simulink model "Target_Control_System"  (R2021b)
settings: Solver=FixedStepDiscrete  StartTime=0.0  StopTime=5  RelTol=1e-3
PreLoadFcn:
  | RTWConfigurationCB('preloadfcn', bdroot);
PostLoadFcn:
  | load('configuration/data_struct.mat');
  | load('configuration/fluxMaps_propMotor.mat');
  | load('configuration/parameterInit_PROP.mat');
  | load('configuration/parameterInit_PUMP.mat');
  | load('configuration/parameterInit_PITCH.mat');
  | load('configuration/parameterInit_TILT.mat');
  | %load('configuration/base_workspace_signal_definition.mat');
  | %load('resolvedatastores_to_baseworkspace_for_faster_simulation.mat');
model workspace (MAT data in the model file):
  SIMULATION_OPTIONS : Simulink.Parameter (value not decoded)
  TARGET_CODE_GEN : Simulink.Parameter (value not decoded)
  TCS_SAMPLE_FREQ_HZ : Simulink.Parameter (value not decoded)
symbols that are objects in the model workspace (value not decoded): TARGET_CODE_GEN, TCS_SAMPLE_FREQ_HZ
undefined symbols (not defined in the file): A_DQ_REF_LPF_INIT__PITCH, A_DQ_REF_LPF_INIT__PROP, A_DQ_REF_LPF_INIT__PUMP, A_DQ_REF_LPF_INIT__TILT, A_OBSERVER_CONFIDENCE_INIT__PITCH, A_OBSERVER_CONFIDENCE_INIT__PROP, A_OBSERVER_CONFIDENCE_INIT__PUMP, A_OBSERVER_CONFIDENCE_INIT__TILT, ACTUATOR_MAX_ANGLE_TRIP__PITCH, ACTUATOR_MIN_ANGLE_TRIP__PITCH, ACTUATOR_POS_SENSOR_INV_DIRECTION__PITCH, ACTUATOR_POS_SENSOR_INV_DIRECTION__TILT, ACTUATOR_POS_SENSOR_OFFSET__PITCH, ACTUATOR_POS_SENSOR_OFFSET__TILT, ADC_scaler1_baseaddr_TILT, ADC_SCALER_FLOAT_TO_FIXPOINT_EXPANSION, ANGLE_ELEC_FROM_SENSOR_OFFSET_INIT__PITCH, ANGLE_ELEC_FROM_SENSOR_OFFSET_INIT__PROP, ANGLE_ELEC_FROM_SENSOR_OFFSET_INIT__PUMP, ANGLE_ELEC_FROM_SENSOR_OFFSET_INIT__TILT, AUTO_CLEAR_FAULTS_ENABLED__PITCH, AUTO_CLEAR_FAULTS_ENABLED__PROP, AUTO_CLEAR_FAULTS_ENABLED__PUMP, AUTO_CLEAR_FAULTS_ENABLED__TILT, AUTO_CLEAR_FAULTS_WAIT_TICKS__PITCH, AUTO_CLEAR_FAULTS_WAIT_TICKS__PROP, AUTO_CLEAR_FAULTS_WAIT_TICKS__PUMP, AUTO_CLEAR_FAULTS_WAIT_TICKS__TILT, AUTO_I_ZERO_IDLE_TICKS__PITCH, AUTO_I_ZERO_IDLE_TICKS__PROP, AUTO_I_ZERO_IDLE_TICKS__PUMP, AUTO_I_ZERO_IDLE_TICKS__TILT, AUTO_I_ZERO_OFFSET_IDC_THRESHOLD__PITCH, AUTO_I_ZERO_OFFSET_IDC_THRESHOLD__PROP, AUTO_I_ZERO_OFFSET_IDC_THRESHOLD__PUMP, AUTO_I_ZERO_OFFSET_IDC_THRESHOLD__TILT, AUTO_I_ZERO_OFFSET_IPH_THRESHOLD__PITCH, AUTO_I_ZERO_OFFSET_IPH_THRESHOLD__PROP, AUTO_I_ZERO_OFFSET_IPH_THRESHOLD__PUMP, AUTO_I_ZERO_OFFSET_IPH_THRESHOLD__TILT, AUTO_SENSORLESS_SWITCHOVER_DISABLE_OMEGA, AUTO_SENSORLESS_SWITCHOVER_ENABLE_OMEGA, AUTO_SENSORLESS_SWITCHOVER_MIN_CONFIDENCE, AUXILIARY_PROTECTION_UNIT_BASEADDR__TILT, blanking_max_error_omega_INIT_PITCH, blanking_max_error_omega_INIT_TILT, blanking_max_error_position_INIT_PITCH, blanking_max_error_position_INIT_TILT, BRUTE_START_I_Q_REF_RAMP_SPEED__PITCH, BRUTE_START_I_Q_REF_RAMP_SPEED__PROP, BRUTE_START_I_Q_REF_RAMP_SPEED__PUMP, BRUTE_START_I_Q_REF_RAMP_SPEED__TILT, CONTROL_LOOP_DT_INIT__PITCH, CONTROL_LOOP_DT_INIT__PROP, CONTROL_LOOP_DT_INIT__PUMP, CONTROL_LOOP_DT_INIT__TILT, CORRECTION_FILTER_SCALE__PITCH, CORRECTION_FILTER_SCALE__PROP, CORRECTION_FILTER_SCALE__PUMP, CORRECTION_FILTER_SCALE__TILT ... (+458)
libraries: simulink x178, Reusables_Lib x24
(part 14 of 47)

== system Target_Control_System/Target_Control_System/MainLoop/propMotor_mainLoop/motorTaskMainFastStep(&oProp)/Lowpass Filtered Quantities for External World - Prop ==
  note: Low-pass filtered quantities for external world
  lpfQuantities : TriggerPort  TriggerType=function-call  VariantControl=Variant
  Constant1 : Constant  Value=0.00008  OutDataTypeStr=single  SampleTime=-1
  Data Store Read17 : DataStoreRead  DataStoreName=oProp  DataStoreElements=oProp.oMot_.oIn_.fId_  IndexOptions=Index vector (dialog)  Indices=1  OutputSizes=1
  Data Store Read18 : DataStoreRead  DataStoreName=oProp  DataStoreElements=oProp.oMot_.oIn_.fIq_  IndexOptions=Index vector (dialog)  Indices=1  OutputSizes=1
  Data Store Read19 : DataStoreRead  DataStoreName=oProp  DataStoreElements=oProp.oMot_.oIn_.fTEstimate_  IndexOptions=Index vector (dialog)  Indices=1  OutputSizes=1
  Data Store Read20 : DataStoreRead  DataStoreName=oProp  DataStoreElements=oProp.oMot_.oOut_.fPowerDcLpf_  IndexOptions=Index vector (dialog)  Indices=1  OutputSizes=1
  Data Store Read21 : DataStoreRead  DataStoreName=oProp  DataStoreElements=oProp.oMot_.oOut_.fPowerDcXlpf_  IndexOptions=Index vector (dialog)  Indices=1  OutputSizes=1
  Data Store Read22 : DataStoreRead  DataStoreName=oProp  DataStoreElements=oProp.oMot_.oIn_.fOmegaEObserverLpf2_  IndexOptions=Index vector (dialog)  Indices=1  OutputSizes=1
  Data Store Read23 : DataStoreRead  DataStoreName=oProp  DataStoreElements=oProp.oMot_.oOut_.fOmegaEObserverXlpf2_  IndexOptions=Index vector (dialog)  Indices=1  OutputSizes=1
  Data Store Read24 : DataStoreRead  DataStoreName=oProp  DataStoreElements=oProp.oMot_.oParam_.fAOmegaXfilter2_  IndexOptions=Index vector (dialog)  Indices=1  OutputSizes=1
  Data Store Read27 : DataStoreRead  DataStoreName=oProp  DataStoreElements=oProp.oMot_.oParam_.fSlowPassFactor_  IndexOptions=Index vector (dialog)  Indices=1  OutputSizes=1
  Data Store Read28 : DataStoreRead  DataStoreName=oProp  DataStoreElements=oProp.oMot_.oIn_.fIPhaseMagnitude_  IndexOptions=Index vector (dialog)  Indices=1  OutputSizes=1
  Data Store Read29 : DataStoreRead  DataStoreName=oProp  DataStoreElements=oProp.oMot_.oState_.fIPhaseMagnitudeLpf_  IndexOptions=Index vector (dialog)  Indices=1  OutputSizes=1
  Data Store Read43 : DataStoreRead  DataStoreName=oProp  DataStoreElements=oProp.oMot_.oOut_.fIdLpf_  IndexOptions=Index vector (dialog)  Indices=1  OutputSizes=1
  Data Store Read44 : DataStoreRead  DataStoreName=oProp  DataStoreElements=oProp.oMot_.oOut_.fIqLpf_  IndexOptions=Index vector (dialog)  Indices=1  OutputSizes=1
  Data Store Read45 : DataStoreRead  DataStoreName=oProp  DataStoreElements=oProp.oMot_.oIn_.oAdcData_.fUdc_  IndexOptions=Index vector (dialog)  Indices=1  OutputSizes=1
  Data Store Read46 : DataStoreRead  DataStoreName=oProp  DataStoreElements=oProp.oMot_.oOut_.fUdcLpf_  IndexOptions=Index vector (dialog)  Indices=1  OutputSizes=1
  Data Store Read47 : DataStoreRead  DataStoreName=oProp  DataStoreElements=oProp.oMot_.oIn_.oAdcData_.fIdc_  IndexOptions=Index vector (dialog)  Indices=1  OutputSizes=1
  Data Store Read48 : DataStoreRead  DataStoreName=oProp  DataStoreElements=oProp.oMot_.oOut_.fIdcLpf_  IndexOptions=Index vector (dialog)  Indices=1  OutputSizes=1
  Data Store Read49 : DataStoreRead  DataStoreName=oProp  DataStoreElements=oProp.oMot_.oIn_.fPowerDc_  IndexOptions=Index vector (dialog)  Indices=1  OutputSizes=1
  Data Store Read50 : DataStoreRead  DataStoreName=oProp  DataStoreElements=oProp.oMot_.oOut_.fPowerDcLpf_  IndexOptions=Index vector (dialog)  Indices=1  OutputSizes=1
  Data Store Read52 : DataStoreRead  DataStoreName=oProp  DataStoreElements=oProp.oMot_.oOut_.fTEstimateLpf_  IndexOptions=Index vector (dialog)  Indices=1  OutputSizes=1
  Data Store Read53 : DataStoreRead  DataStoreName=oProp  DataStoreElements=oProp.oMot_.oState_.oRampDataIqRef_.fRampOut_  IndexOptions=Index vector (dialog)  Indices=1  OutputSizes=1
  Data Store Read54 : DataStoreRead  DataStoreName=oProp  DataStoreElements=oProp.oMot_.oOut_.fIqRefRampOutLpf_  IndexOptions=Index vector (dialog)  Indices=1  OutputSizes=1
  Data Store Read55 : DataStoreRead  DataStoreName=oProp  DataStoreElements=oProp.oMot_.oParam_.fADqRefLpf_  IndexOptions=Index vector (dialog)  Indices=1  OutputSizes=1
  Data Store Read56 : DataStoreRead  DataStoreName=oProp  DataStoreElements=oProp.oMot_.oIn_.fIdRefTotal_  IndexOptions=Index vector (dialog)  Indices=1  OutputSizes=1
  Data Store Read57 : DataStoreRead  DataStoreName=oProp  DataStoreElements=oProp.oMot_.oOut_.fIdRefLpf_  IndexOptions=Index vector (dialog)  Indices=1  OutputSizes=1
  Data Store Read58 : DataStoreRead  DataStoreName=oProp  DataStoreElements=oProp.oMot_.oIn_.fUqRef_  IndexOptions=Index vector (dialog)  Indices=1  OutputSizes=1
  Data Store Read59 : DataStoreRead  DataStoreName=oProp  DataStoreElements=oProp.oMot_.oOut_.fUqRefLpf_  IndexOptions=Index vector (dialog)  Indices=1  OutputSizes=1
  Data Store Read60 : DataStoreRead  DataStoreName=oProp  DataStoreElements=oProp.oMot_.oIn_.fUdRef_  IndexOptions=Index vector (dialog)  Indices=1  OutputSizes=1
  Data Store Read62 : DataStoreRead  DataStoreName=oProp  DataStoreElements=oProp.oMot_.oOut_.fUdRefLpf_  IndexOptions=Index vector (dialog)  Indices=1  OutputSizes=1
  Data Store Write2 : DataStoreWrite  DataStoreName=oProp  DataStoreElements=oProp.oMot_.oOut_.fPowerDcXlpf_  IndexOptions=Index vector (dialog)  Indices=1  OutputSizes=1
  Data Store Write20 : DataStoreWrite  DataStoreName=oProp  DataStoreElements=oProp.oMot_.oState_.fIPhaseMagnitudeLpf_  IndexOptions=Index vector (dialog)  Indices=1  OutputSizes=1
  Data Store Write21 : DataStoreWrite  DataStoreName=oProp  DataStoreElements=oProp.oMot_.oOut_.fIdLpf_  IndexOptions=Index vector (dialog)  Indices=1  OutputSizes=1
  Data Store Write22 : DataStoreWrite  DataStoreName=oProp  DataStoreElements=oProp.oMot_.oOut_.fIqLpf_  IndexOptions=Index vector (dialog)  Indices=1  OutputSizes=1
  Data Store Write24 : DataStoreWrite  DataStoreName=oProp  DataStoreElements=oProp.oMot_.oOut_.fUdcLpf_  IndexOptions=Index vector (dialog)  Indices=1  OutputSizes=1
  Data Store Write25 : DataStoreWrite  DataStoreName=oProp  DataStoreElements=oProp.oMot_.oOut_.fIdcLpf_  IndexOptions=Index vector (dialog)  Indices=1  OutputSizes=1
  Data Store Write28 : DataStoreWrite  DataStoreName=oProp  DataStoreElements=oProp.oMot_.oOut_.fPowerDcLpf_  IndexOptions=Index vector (dialog)  Indices=1  OutputSizes=1
  Data Store Write29 : DataStoreWrite  DataStoreName=oProp  DataStoreElements=oProp.oMot_.oOut_.fTEstimateLpf_  IndexOptions=Index vector (dialog)  Indices=1  OutputSizes=1
  Data Store Write3 : DataStoreWrite  DataStoreName=oProp  DataStoreElements=oProp.oMot_.oOut_.fOmegaEObserverXlpf2_  IndexOptions=Index vector (dialog)  Indices=1  OutputSizes=1
  Data Store Write30 : DataStoreWrite  DataStoreName=oProp  DataStoreElements=oProp.oMot_.oOut_.fIqRefRampOutLpf_  IndexOptions=Index vector (dialog)  Indices=1  OutputSizes=1
  Data Store Write31 : DataStoreWrite  DataStoreName=oProp  DataStoreElements=oProp.oMot_.oOut_.fIdRefLpf_  IndexOptions=Index vector (dialog)  Indices=1  OutputSizes=1
  Data Store Write32 : DataStoreWrite  DataStoreName=oProp  DataStoreElements=oProp.oMot_.oOut_.fUqRefLpf_  IndexOptions=Index vector (dialog)  Indices=1  OutputSizes=1
  Data Store Write34 : DataStoreWrite  DataStoreName=oProp  DataStoreElements=oProp.oMot_.oOut_.fUdRefLpf_  IndexOptions=Index vector (dialog)  Indices=1  OutputSizes=1
  Divide{8..20} (13 alike) : Product  Inputs=**
  Sum{4..5,7,10..11,13,15,18,20..22,25,29} (13 alike) : Sum  Inputs=|+-
  Sum{3,6,8..9,12,14,16..17,19,24,26,30..31} (13 alike) : Sum  Inputs=|++
  wires:
  Sum10/1 -> Divide13/2
  Data Store Read22/1 -> Sum22/1
  Divide12/1 -> Sum9/1
  Sum3/1 -> Data Store Write20/1
  Divide20/1 -> Sum24/1
  Sum13/1 -> Divide12/2
  Sum19/1 -> Data Store Write31/1
  Data Store Read46/1 -> Sum13/2, Sum9/2
  Divide17/1 -> Sum30/1
  Data Store Read43/1 -> Sum4/2, Sum6/2
  Sum18/1 -> Divide15/2
  Sum22/1 -> Divide18/2
  Data Store Read23/1 -> Sum26/2, Sum22/2
  Divide9/1 -> Sum6/1
  Data Store Read24/1 -> Divide18/1
  Data Store Read18/1 -> Sum5/1
  Sum8/1 -> Data Store Write22/1
  Data Store Read44/1 -> Sum5/2, Sum8/2
  Data Store Read28/1 -> Sum7/1
  Data Store Read21/1 -> Sum24/2, Sum21/2
  Sum9/1 -> Data Store Write24/1
  Sum5/1 -> Divide10/2
  Sum4/1 -> Divide9/2
  Data Store Read55/1 -> Divide15/1, Divide16/1, Divide19/1, Divide17/1
  Sum15/1 -> Divide14/2
  Divide8/1 -> Sum3/1
  Sum29/1 -> Divide17/2
  Data Store Read27/1 -> Divide8/1, Divide9/1, Divide10/1, Divide12/1, Divide13/1, Divide14/1, Divide11/1
  Sum11/1 -> Divide11/2
  Sum14/1 -> Data Store Write28/1
  Data Store Read20/1 -> Sum21/1
  Data Store Read54/1 -> Sum18/2, Sum17/2
  Data Store Read56/1 -> Sum20/1
  Divide18/1 -> Sum26/1
  Constant1/1 -> Divide20/1
  Sum30/1 -> Data Store Write32/1
  Data Store Read49/1 -> Sum11/1
  Sum25/1 -> Divide19/2
  Data Store Read45/1 -> Sum13/1
  Divide15/1 -> Sum17/1
  Divide14/1 -> Sum16/1
  Sum26/1 -> Data Store Write3/1
  Sum24/1 -> Data Store Write2/1
  Data Store Read17/1 -> Sum4/1
  Divide13/1 -> Sum12/1
  Sum20/1 -> Divide16/2
  Data Store Read62/1 -> Sum25/2, Sum31/2
  Divide16/1 -> Sum19/1
  Data Store Read60/1 -> Sum25/1
  Data Store Read57/1 -> Sum20/2, Sum19/2
  Sum21/1 -> Divide20/2
  Data Store Read48/1 -> Sum12/2, Sum10/2
  Sum16/1 -> Data Store Write29/1
  Divide11/1 -> Sum14/1
  Data Store Read19/1 -> Sum15/1
  Sum6/1 -> Data Store Write21/1
  Sum7/1 -> Divide8/2
  Data Store Read29/1 -> Sum7/2, Sum3/2
  Data Store Read50/1 -> Sum14/2, Sum11/2
  Divide10/1 -> Sum8/1
  Sum12/1 -> Data Store Write25/1
  Data Store Read59/1 -> Sum29/2, Sum30/2
  Data Store Read47/1 -> Sum10/1
  Data Store Read52/1 -> Sum16/2, Sum15/2
  Sum17/1 -> Data Store Write30/1
  Data Store Read53/1 -> Sum18/1
  Sum31/1 -> Data Store Write34/1
  Divide19/1 -> Sum31/1
  Data Store Read58/1 -> Sum29/1

== system Target_Control_System/Target_Control_System/MainLoop/propMotor_mainLoop/motorTaskMainFastStep(&oProp)/Observer Confidence - Prop ==
  note: Observer confidence
      | // Two contributions, each adding 1/3 to give a value in range 0.0-1.0:
      | 	//  1. Magnitude of estimated flux relative to nominal flux (perhaps not for induction motors)
      | 	//  2. The relative noise on the estimated speed
  observerConfidence : TriggerPort  TriggerType=function-call  VariantControl=Variant
  Abs2 : Abs  OutDataTypeStr=single
  Abs3 : Abs  OutDataTypeStr=single
  Abs5 : Abs  OutDataTypeStr=single
  Add10 : Sum  Inputs=|-+
  Add11 : Sum
  Add2 : Sum  Inputs=+-
  Add7 : Sum  Inputs=|+-
  Add8 : Sum  Inputs=|-+
  Add9 : Sum  Inputs=|-+
  Constant14 : Constant  OutDataTypeStr=single  SampleTime=-1
  Data Store Read1 : DataStoreRead  DataStoreName=oProp  DataStoreElements=oProp.oMot_.oParam_.fAObserverConfidence_  IndexOptions=Index vector (dialog)  Indices=1  OutputSizes=1
  Data Store Read37 : DataStoreRead  DataStoreName=oProp  DataStoreElements=oProp.oMot_.oIn_.fOmegaEObserverLpf2_  IndexOptions=Index vector (dialog)  Indices=1  OutputSizes=1
  Data Store Read4 : DataStoreRead  DataStoreName=oProp  DataStoreElements=oProp.oMot_.oIn_.fFluxMainMagnitudeLpf_  IndexOptions=Index vector (dialog)  Indices=1  OutputSizes=1
  Data Store Read61 : DataStoreRead  DataStoreName=oProp  DataStoreElements=oProp.oMot_.oIn_.fOmegaEObserverRaw2_  IndexOptions=Index vector (dialog)  Indices=1  OutputSizes=1
  Data Store Read83 : DataStoreRead  DataStoreName=oProp  DataStoreElements=oProp.oMot_.oParam_.fMainFluxNominal_  IndexOptions=Index vector (dialog)  Indices=1  OutputSizes=1
  Data Store Write33 : DataStoreWrite  DataStoreName=oProp  DataStoreElements=oProp.oMot_.oState_.fObserverConfidence_  IndexOptions=Index vector (dialog)  Indices=1  OutputSizes=1
  Divide1 : Product  Inputs=*/
  Divide2 : Product  Inputs=*/
  Gain11 : Gain  Gain=0.83
  Gain5 : Gain  Gain=0.4
  Half : Constant  Value=0.5  OutDataTypeStr=single  SampleTime=-1
  Half1 : Constant  Value=0.5  OutDataTypeStr=single  SampleTime=-1
  IIR : Subsystem
  Saturation2 : Saturate  UpperLimit=1.25  LowerLimit=-inf
  Saturation3 : Saturate  UpperLimit=0.6  LowerLimit=-inf
  Switch3 : Switch  Criteria=u2 > Threshold  Threshold=0.5
  Zero8 : Constant  Value=0  OutDataTypeStr=Inherit: Inherit via back propagation  SampleTime=-1
  isNaN : RelationalOperator  Operator=isNaN  OutDataTypeStr=boolean  RndMeth=Simplest
  wires:
  Data Store Read1/1 -> IIR/3(K), Add2/2
  Abs5/1 -> Divide2/2
  Add11/1 -> isNaN/1, Switch3/3  "fObserverConfidence_"
  Data Store Read83/1 -> Divide1/2, Add7/2
  Gain5/1 -> Add8/1
  Add2/1 -> IIR/2(1-K)
  Half1/1 -> Add10/2
  isNaN/1 -> Switch3/2
  Abs3/1 -> Divide2/1
  Gain11/1 -> Add10/1
  Divide1/1 -> Saturation2/1
  Switch3/1 -> IIR/1(In)
  Zero8/1 -> Switch3/1
  Abs2/1 -> Divide1/1
  Data Store Read37/1 -> Add9/2, Abs5/1
  Half/1 -> Add8/2
  Saturation2/1 -> Gain5/1
  Constant14/1 -> Add2/1
  Data Store Read61/1 -> Add9/1
  Add9/1 -> Abs3/1
  Divide2/1 -> Saturation3/1
  IIR/1(Out) -> Data Store Write33/1
  Add7/1 -> Abs2/1
  Add8/1 -> Add11/1
  Add10/1 -> Add11/2
  Saturation3/1 -> Gain11/1
  Data Store Read4/1 -> Add7/1

== system Target_Control_System/Target_Control_System/MainLoop/propMotor_mainLoop/motorTaskMainFastStep(&oProp)/PWM for Simulation ==
  Enable : EnablePort
  Constant : Constant  OutDataTypeStr=uint32  SampleTime=-1
  Constant1 : Constant  Value=0  OutDataTypeStr=uint32  SampleTime=-1
  Data Store Read1 : DataStoreRead  DataStoreName=oProp  DataStoreElements=oProp.oIsr_.oState_.iPwmUpdated_  IndexOptions=Index vector (dialog)  Indices=1  OutputSizes=1
  Data Store Write18 : DataStoreWrite  DataStoreName=oProp  DataStoreElements=oProp.oIsr_.oOut_.uiPwmSetByIsr_  IndexOptions=Index vector (dialog)  Indices=1  OutputSizes=1
  NOT : Logic  Operator=NOT  AllPortsSameDT=off  OutDataTypeStr=boolean
  Scope : Scope
  Subsystem : Subsystem
  Subsystem1 : Subsystem
  Switch1 : Switch  Criteria=u2 > Threshold
  Switch2 : Switch  Criteria=u2 > Threshold
  Motor : Outport
  wires:
  NOT/1 -> Subsystem1/Enable
  Subsystem1/1(propMotor_PWMticks) -> Switch1/3
  Subsystem/1(propMotor_PWMticks) -> Switch1/1
  Constant1/1 -> Switch2/3
  Constant/1 -> Switch2/1
  Switch2/1 -> Data Store Write18/1
  Switch1/1 -> Motor/1  "propMotor_PWMticks"
  Data Store Read1/1 -> Subsystem/Enable, Switch1/2, NOT/1, Scope/1, Switch2/2

== system Target_Control_System/Target_Control_System/MainLoop/propMotor_mainLoop/motorTaskMainFastStep(&oProp)/motorTaskManagePwmRequestFlags() ==
  motorTaskManagePwmRequestFlags : TriggerPort  TriggerType=function-call  VariantControl=Variant
  Constant : Constant  Value=0  OutDataTypeStr=uint32  SampleTime=-1
  Data Store Read : DataStoreRead  DataStoreName=oProp  DataStoreElements=oProp.oMot_.oIn_.uiPwmSetByIsr_  IndexOptions=Index vector (dialog)  Indices=1  OutputSizes=1
  Data Store Read1 : DataStoreRead  DataStoreName=oProp  DataStoreElements=oProp.oMot_.oOut_.uiPwmRequestFromMain_  IndexOptions=Index vector (dialog)  Indices=1  OutputSizes=1
  Data Store Write : DataStoreWrite  DataStoreName=oProp  DataStoreElements=oProp.oMot_.oOut_.uiPwmRequestFromMain_  IndexOptions=Index vector (dialog)  Indices=1  OutputSizes=1
  Switch : Switch  Criteria=u2 > Threshold  OutDataTypeStr=uint32
  wires:
  Data Store Read1/1 -> Switch/3
  Constant/1 -> Switch/1
  Switch/1 -> Data Store Write/1
  Data Store Read/1 -> Switch/2

== system Target_Control_System/Target_Control_System/MainLoop/propMotor_mainLoop/motorTaskMainFastStep(&oProp)/resetFlag_uiDataFromIsrToMainUpdated ==
  resetFlag_uiDataFromIsrToMainUpdated : TriggerPort  TriggerType=function-call  VariantControl=Variant
  Constant : Constant  Value=0  OutDataTypeStr=uint32  SampleTime=-1
  Data Store Write9 : DataStoreWrite  DataStoreName=oProp  DataStoreElements=oProp.oMot_.oIn_.uiDataFromIsrToMainUpdated_  IndexOptions=Index vector (dialog)  Indices=1  OutputSizes=1
  wires:
  Constant/1 -> Data Store Write9/1

== system Target_Control_System/Target_Control_System/MainLoop/pumpMotor_mainLoop/Decimation gate A for 200 Hz Pump/Current offset nulling ==
  note: Try to perform current sensor offset nulling at least once as soon as possible:
      | (Subsequent nulling steps are performed only once the drive has been idle for a while)
  function : TriggerPort  TriggerType=function-call  VariantControl=Variant
  Constant2 : Constant  Value=0  OutDataTypeStr=uint32  SampleTime=-1
  Data Store Read2 : DataStoreRead  DataStoreName=oPump  DataStoreElements=oPump.oMot_.oState_.uiCurrentOffsetNullingPerformed_  IndexOptions=Index vector (dialog)  Indices=1  OutputSizes=1
  GreaterThan1 : RelationalOperator  Operator=>  OutDataTypeStr=boolean  RndMeth=Simplest
  NOT : Logic  Operator=NOT  IconShape=distinctive  AllPortsSameDT=off  OutDataTypeStr=boolean
  initiateOffsetNulling(&oPump) : Subsystem  TreatAsAtomicUnit=on
  wires:
  NOT/1 -> initiateOffsetNulling(&oPump)/Enable
  GreaterThan1/1 -> NOT/1
  Constant2/1 -> GreaterThan1/2
  Data Store Read2/1 -> GreaterThan1/1

== system Target_Control_System/Target_Control_System/MainLoop/pumpMotor_mainLoop/Decimation gate A for 200 Hz Pump/Subsystem ==
  Idle_Controller : TriggerPort  TriggerType=function-call  VariantControl=Variant
  AND7 : Logic  AllPortsSameDT=off  OutDataTypeStr=boolean
  Data Store Read1 : DataStoreRead  DataStoreName=oPump  DataStoreElements=oPump.oMot_.oParam_.oPiDataIdleCtrl_.fState_  IndexOptions=Index vector (dialog)  Indices=1  OutputSizes=1
  Data Store Read2 : DataStoreRead  DataStoreName=oPump  DataStoreElements=oPump.oMot_.oParam_.fRpmBlankingUnblankConfidence_  IndexOptions=Index vector (dialog)  Indices=1  OutputSizes=1
  Data Store Read25 : DataStoreRead  DataStoreName=oPump  DataStoreElements=oPump.oMot_.oState_.uiDriveState_  IndexOptions=Index vector (dialog)  Indices=1  OutputSizes=1
  Data Store Read3 : DataStoreRead  DataStoreName=oPump  DataStoreElements=oPump.oMot_.oParam_.fRpmBlankingBlankConfidence_  IndexOptions=Index vector (dialog)  Indices=1  OutputSizes=1
  Data Store Read32 : DataStoreRead  DataStoreName=oPump  DataStoreElements=oPump.oMot_.oState_.fObserverConfidence_  IndexOptions=Index vector (dialog)  Indices=1  OutputSizes=1
  Data Store Read51 : DataStoreRead  DataStoreName=oPump  DataStoreElements=oPump.oMot_.oState_.uiDriveState_  IndexOptions=Index vector (dialog)  Indices=1  OutputSizes=1
  Data Store Read65 : DataStoreRead  DataStoreName=oPump  DataStoreElements=oPump.oMot_.oOut_.fOmegaEObserverXlpf2_  IndexOptions=Index vector (dialog)  Indices=1  OutputSizes=1
  Data Store Read66 : DataStoreRead  DataStoreName=oPump  DataStoreElements=oPump.oMot_.oState_.fIdleCtrlOmegaEMin_  IndexOptions=Index vector (dialog)  Indices=1  OutputSizes=1
  Data Store Read67 : DataStoreRead  DataStoreName=oPump  DataStoreElements=oPump.oMot_.oParam_.oPiDataIdleCtrl_.oParameter_.fKp_  IndexOptions=Index vector (dialog)  Indices=1  OutputSizes=1
  Data Store Read69 : DataStoreRead  DataStoreName=oPump  DataStoreElements=oPump.oMot_.oParam_.oPiDataIdleCtrl_.oParameter_.fKi_  IndexOptions=Index vector (dialog)  Indices=1  OutputSizes=1
  Data Store Read70 : DataStoreRead  DataStoreName=oPump  DataStoreElements=oPump.oMot_.oParam_.oPiDataIdleCtrl_.oParameter_.fIntMax_  IndexOptions=Index vector (dialog)  Indices=1  OutputSizes=1
  Data Store Read94 : DataStoreRead  DataStoreName=oPump  DataStoreElements=oPump.oMot_.oParam_.oPiDataIdleCtrl_.oParameter_.fOutMax_  IndexOptions=Index vector (dialog)  Indices=1  OutputSizes=1
  Data Store Read95 : DataStoreRead  DataStoreName=oPump  DataStoreElements=oPump.oMot_.oParam_.oPiDataIdleCtrl_.oParameter_.fLoopDt_  IndexOptions=Index vector (dialog)  Indices=1  OutputSizes=1
  Data Store Write5 : DataStoreWrite  DataStoreName=oPump  DataStoreElements=oPump.oMot_.oState_.iRpmBlankingActive_  IndexOptions=Index vector (dialog)  Indices=1  OutputSizes=1
  Equal12 : RelationalOperator  Operator===  OutDataTypeStr=boolean  RndMeth=Simplest
  Equal16 : RelationalOperator  Operator=~=  OutDataTypeStr=boolean  RndMeth=Simplest
  Equal17 : RelationalOperator  Operator=~=  OutDataTypeStr=boolean  RndMeth=Simplest
  NOT : Logic  Operator=NOT  AllPortsSameDT=off  OutDataTypeStr=boolean
  OR (Never blank in state 200)1 : Logic  Operator=OR  AllPortsSameDT=off  OutDataTypeStr=boolean
  Subsystem : Subsystem
  Switch2 : Switch  Criteria=u2 > Threshold  Threshold=0.5  OutDataTypeStr=int32
  Zero18 : Constant  Value=0  OutDataTypeStr=single  SampleTime=-1
  Zero19 : Constant  OutDataTypeStr=single  SampleTime=-1
  Zero8 : Constant  Value=0  OutDataTypeStr=single  SampleTime=-1
  const12 : Constant  Value=200  OutDataTypeStr=uint32  SampleTime=-1
  const13 : Constant  Value=211  OutDataTypeStr=uint32  SampleTime=-1
  const14 : Constant  Value=212  OutDataTypeStr=uint32  SampleTime=-1
  greater1 : RelationalOperator  Operator=>  OutDataTypeStr=boolean  RndMeth=Simplest
  piControllerStep_Idle_Controller : Subsystem  SystemSampleTime=1/200
  smaller1 : RelationalOperator  Operator=<  OutDataTypeStr=boolean  RndMeth=Simplest
  wires:
  smaller1/1 -> Switch2/3
  Switch2/1 -> Data Store Write5/1
  Zero8/1 -> Switch2/1
  Data Store Read32/1 -> smaller1/1, greater1/1
  const12/1 -> Equal12/2
  Data Store Read2/1 -> greater1/2
  Equal12/1 -> OR (Never blank in state 200)1/1
  Data Store Read3/1 -> smaller1/2
  greater1/1 -> OR (Never blank in state 200)1/2
  Data Store Read25/1 -> Equal12/1
  OR (Never blank in state 200)1/1 -> Switch2/2
  NOT/1 -> Subsystem/Enable
  Data Store Read1/1 -> piControllerStep_Idle_Controller/11(fState)
  const13/1 -> Equal16/1
  Data Store Read67/1 -> piControllerStep_Idle_Controller/3(fKp)
  Data Store Read94/1 -> piControllerStep_Idle_Controller/8(fOutMax)
  Data Store Read66/1 -> piControllerStep_Idle_Controller/2(fTarget)
  Zero19/1 -> piControllerStep_Idle_Controller/5(fScale)
  Data Store Read70/1 -> piControllerStep_Idle_Controller/7(fIntMax)
  Data Store Read95/1 -> piControllerStep_Idle_Controller/6(fLoopDt)
  Data Store Read69/1 -> piControllerStep_Idle_Controller/4(fKi)
  Data Store Read51/1 -> Equal16/2, Equal17/1
  Equal17/1 -> AND7/2
  Zero18/1 -> piControllerStep_Idle_Controller/9(fIntMin), piControllerStep_Idle_Controller/10(fOutMin)
  AND7/1 -> piControllerStep_Idle_Controller/Enable, NOT/1
  const14/1 -> Equal17/2
  Data Store Read65/1 -> piControllerStep_Idle_Controller/1(fActual)
  Equal16/1 -> AND7/1

== system Target_Control_System/Target_Control_System/MainLoop/pumpMotor_mainLoop/Decimation gate for 5000 Hz Pump/motorTaskProcessExternalSetpoints(&oPump) ==
  note: // Do not set certain variables during auto forced angle start or resistance measurement // This whole code below should be cleaned up, probably a switch case tied to the state machine.
      | // The different modes, (position control, speed control, current control) should get different state numbers to facilitate this.
  note: // Take externally requested setpoints (already set in the 'in' struct) and apply them (after sanitizing) to the right place in the control loop, also depending on the state that the drive is in.
  motorTaskProcessExternalSetpoints : TriggerPort  TriggerType=function-call  VariantControl=Variant
  Function-Call Generator : simulink/Ports & Subsystems/Function-Call Generator  sample_time=-1  numberOfIterations=1  DisallowWideOutput=off
  Function-Call Split1 : FunctionCallSplit  NumOutputPorts=2
  Function-Call Split10 : FunctionCallSplit  NumOutputPorts=2
  Subsystem1 : Subsystem
  Subsystem2 : Subsystem
  Subsystem3 : Subsystem
  wires:
  Function-Call Split1/2 -> Subsystem3/Trigger
  Function-Call Split10/2 -> Function-Call Split1/1
  Function-Call Split1/1 -> Subsystem2/Trigger
  Function-Call Split10/1 -> Subsystem1/Trigger
  Function-Call Generator/1 -> Function-Call Split10/1

== system Target_Control_System/Target_Control_System/MainLoop/pumpMotor_mainLoop/motorTaskMainFastStep(&oPump)/Control Loops - Pump ==
  note: mdl_fIdFluxWeakeningSetpoint_
  note: ---------- runFluxWeakeningCurrentCalculation ------------
      | 	// This function calculates how much flux weakening current is needed to keep the modulation index below full scale.
      | 	// It uses positive numbers exclusively for ease of reading & reasoning; the calling function
      | 	// will have to include a minus sign somewhere to turn it into negative d-current.
  note: // If the speed is too low, just return zero. // This is a simple safety catch to prevent injecting d current when there should be no need for it.
  controlLoops : TriggerPort  TriggerType=function-call  VariantControl=Variant
  AND8 : Logic  AllPortsSameDT=off  OutDataTypeStr=boolean
  Abs6 : Abs  Commented=on
  Add12 : Sum  Commented=on  Inputs=+-
  Constant3 : Constant  Commented=on  Value=0  OutDataTypeStr=single  SampleTime=-1
  Data Store Read1 : DataStoreRead  DataStoreName=oPump  DataStoreElements=oPump.oMot_.oState_.oRampDataFluxMstrAngFrcd2clsdSmoothn_.oParam_.fTimestepS_  IndexOptions=Index vector (dialog)  Indices=1  OutputSizes=1
  Data Store Read10 : DataStoreRead  DataStoreName=oPump  DataStoreElements=oPump.oMot_.oState_.oRampDataOmegaERef_.oParam_.fUpslope_  IndexOptions=Index vector (dialog)  Indices=1  OutputSizes=1
  Data Store Read100 : DataStoreRead  DataStoreName=oPump  DataStoreElements=oPump.oMot_.oState_.fForcedAngleStartOrigOmegaRamp_  IndexOptions=Index vector (dialog)  Indices=1  OutputSizes=1
  Data Store Read104 : DataStoreRead  DataStoreName=oPump  DataStoreElements=oPump.oMot_.oState_.fForcedAngleStartOrigIRamp_  IndexOptions=Index vector (dialog)  Indices=1  OutputSizes=1
  Data Store Read105 : DataStoreRead  DataStoreName=oPump  DataStoreElements=oPump.oMot_.oState_.oRampDataIqRef_.oParam_.fUpslope_  IndexOptions=Index vector (dialog)  Indices=1  OutputSizes=1
  Data Store Read106 : DataStoreRead  DataStoreName=oPump  DataStoreElements=oPump.oMot_.oParam_.fForcedAngleOmegaEHandoff_  IndexOptions=Index vector (dialog)  Indices=1  OutputSizes=1
  Data Store Read15 : DataStoreRead  DataStoreName=oPump  DataStoreElements=oPump.oMot_.oState_.oRampDataFluxMasterAngleOffset_.oParam_.fUpslope_  IndexOptions=Index vector (dialog)  Indices=1  OutputSizes=1
  Data Store Read2 : DataStoreRead  DataStoreName=oPump  DataStoreElements=oPump.oMot_.oState_.oRampDataFluxMstrAngFrcd2clsdSmoothn_.oParam_.fUpslope_  IndexOptions=Index vector (dialog)  Indices=1  OutputSizes=1
  Data Store Read3 : DataStoreRead  DataStoreName=oPump  DataStoreElements=oPump.oMot_.oState_.oRampDataFluxMstrAngFrcd2clsdSmoothn_.oParam_.fDownslope_  IndexOptions=Index vector (dialog)  Indices=1  OutputSizes=1
  Data Store Read31 : DataStoreRead  Commented=on  DataStoreName=oPump  DataStoreElements=oPump.oMot_.oIn_.fOmegaEObserverLpf2_  IndexOptions=Index vector (dialog)  Indices=1  OutputSizes=1
  Data Store Read4 : DataStoreRead  DataStoreName=oPump  DataStoreElements=oPump.oMot_.oState_.oRampDataFluxMasterAngleOffset_.fSetpoint_  IndexOptions=Index vector (dialog)  Indices=1  OutputSizes=1
  Data Store Read5 : DataStoreRead  Commented=on  DataStoreName=oPump  DataStoreElements=oPump.oMot_.oState_.fIdExternalSetpoint_  IndexOptions=Index vector (dialog)  Indices=1  OutputSizes=1
  Data Store Read6 : DataStoreRead  DataStoreName=oPump  DataStoreElements=oPump.oMot_.oState_.oRampDataIqRef_.fRampOut_  IndexOptions=Index vector (dialog)  Indices=1  OutputSizes=1
  Data Store Read62 : DataStoreRead  DataStoreName=oPump  DataStoreElements=oPump.oMot_.oState_.uiSpeedControllerActive_  IndexOptions=Index vector (dialog)  Indices=1  OutputSizes=1
  Data Store Read63 : DataStoreRead  DataStoreName=oPump  DataStoreElements=oPump.oMot_.oState_.oRampDataFluxMasterAngleOffset_.oParam_.fDownslope_  IndexOptions=Index vector (dialog)  Indices=1  OutputSizes=1
  Data Store Read64 : DataStoreRead  DataStoreName=oPump  DataStoreElements=oPump.oMot_.oState_.oRampDataFluxMasterAngleOffset_.oParam_.fTimestepS_  IndexOptions=Index vector (dialog)  Indices=1  OutputSizes=1
  Data Store Read65 : DataStoreRead  Commented=on  DataStoreName=oPump  DataStoreElements=oPump.oMot_.oParam_.fFluxWeakeningMinimumOmegaE_  IndexOptions=Index vector (dialog)  Indices=1  OutputSizes=1
  Data Store Read68 : DataStoreRead  DataStoreName=oPump  DataStoreElements=oPump.oMot_.oState_.oRampDataIdRef_.oParam_.fTimestepS_  IndexOptions=Index vector (dialog)  Indices=1  OutputSizes=1
  Data Store Read71 : DataStoreRead  DataStoreName=oPump  DataStoreElements=oPump.oMot_.oState_.oRampDataIqRef_.oParam_.fTimestepS_  IndexOptions=Index vector (dialog)  Indices=1  OutputSizes=1
  Data Store Read73 : DataStoreRead  DataStoreName=oPump  DataStoreElements=oPump.oMot_.oState_.oRampDataIqRef_.oParam_.fUpslope_  IndexOptions=Index vector (dialog)  Indices=1  OutputSizes=1
  Data Store Read76 : DataStoreRead  DataStoreName=oPump  DataStoreElements=oPump.oMot_.oState_.oRampDataIqRef_.oParam_.fDownslope_  IndexOptions=Index vector (dialog)  Indices=1  OutputSizes=1
  Data Store Read77 : DataStoreRead  DataStoreName=oPump  DataStoreElements=oPump.oMot_.oState_.oRampDataOmegaERef_.oParam_.fTimestepS_  IndexOptions=Index vector (dialog)  Indices=1  OutputSizes=1
  Data Store Read78 : DataStoreRead  DataStoreName=oPump  DataStoreElements=oPump.oMot_.oState_.oRampDataOmegaERef_.oParam_.fUpslope_  IndexOptions=Index vector (dialog)  Indices=1  OutputSizes=1
  Data Store Read80 : DataStoreRead  DataStoreName=oPump  DataStoreElements=oPump.oMot_.oParam_.fIqSetpointMax_  IndexOptions=Index vector (dialog)  Indices=1  OutputSizes=1
  Data Store Read81 : DataStoreRead  DataStoreName=oPump  DataStoreElements=oPump.oMot_.oParam_.fDynILimIntegratorLeakageFactor_  IndexOptions=Index vector (dialog)  Indices=1  OutputSizes=1
  Data Store Read82 : DataStoreRead  DataStoreName=oPump  DataStoreElements=oPump.oMot_.oState_.fIqRefBeforeRamp_  IndexOptions=Index vector (dialog)  Indices=1  OutputSizes=1
  Data Store Read84 : DataStoreRead  DataStoreName=oPump  DataStoreElements=oPump.oMot_.oState_.fIdleCtrlCurrent_  IndexOptions=Index vector (dialog)  Indices=1  OutputSizes=1
  Data Store Read85 : DataStoreRead  DataStoreName=oPump  DataStoreElements=oPump.oMot_.oState_.oRampDataIdRef_.oParam_.fUpslope_  IndexOptions=Index vector (dialog)  Indices=1  OutputSizes=1
  Data Store Read86 : DataStoreRead  DataStoreName=oPump  DataStoreElements=oPump.oMot_.oState_.oRampDataIdRef_.oParam_.fDownslope_  IndexOptions=Index vector (dialog)  Indices=1  OutputSizes=1
  Data Store Read87 : DataStoreRead  DataStoreName=oPump  DataStoreElements=oPump.oMot_.oState_.oRampDataOmegaERef_.oParam_.fDownslope_  IndexOptions=Index vector (dialog)  Indices=1  OutputSizes=1
  Data Store Write18 : DataStoreWrite  DataStoreName=oPump  DataStoreElements=oPump.oMot_.oState_.oRampDataIqRef_.fRampOut_  IndexOptions=Index vector (dialog)  Indices=1  OutputSizes=1
  Data Store Write19 : DataStoreWrite  DataStoreName=oPump  DataStoreElements=oPump.oMot_.oState_.oRampDataIqRef_.fSetpoint_  IndexOptions=Index vector (dialog)  Indices=1  OutputSizes=1
  Data Store Write2 : DataStoreWrite  DataStoreName=oPump  DataStoreElements=oPump.oMot_.oState_.oRampDataFluxMstrAngFrcd2clsdSmoothn_.fRampOut_  IndexOptions=Index vector (dialog)  Indices=1  OutputSizes=1
  Data Store Write21 : DataStoreWrite  DataStoreName=oPump  DataStoreElements=oPump.oMot_.oState_.oRampDataIdRef_.fRampOut_  IndexOptions=Index vector (dialog)  Indices=1  OutputSizes=1
  Data Store Write22 : DataStoreWrite  DataStoreName=oPump  DataStoreElements=oPump.oMot_.oState_.oRampDataIdRef_.fRampOutDdt_  IndexOptions=Index vector (dialog)  Indices=1  OutputSizes=1
  Data Store Write23 : DataStoreWrite  DataStoreName=oPump  DataStoreElements=oPump.oMot_.oState_.oRampDataOmegaERef_.fRampOut_  IndexOptions=Index vector (dialog)  Indices=1  OutputSizes=1
  Data Store Write26 : DataStoreWrite  DataStoreName=oPump  DataStoreElements=oPump.oMot_.oState_.oRampDataIqRef_.fRampOutDdt_  IndexOptions=Index vector (dialog)  Indices=1  OutputSizes=1
  Data Store Write27 : DataStoreWrite  DataStoreName=oPump  DataStoreElements=oPump.oMot_.oState_.oRampDataOmegaERef_.fRampOutDdt_  IndexOptions=Index vector (dialog)  Indices=1  OutputSizes=1
  Data Store Write3 : DataStoreWrite  DataStoreName=oPump  DataStoreElements=oPump.oMot_.oState_.oRampDataFluxMstrAngFrcd2clsdSmoothn_.fRampOutDdt_  IndexOptions=Index vector (dialog)  Indices=1  OutputSizes=1
  Data Store Write35 : DataStoreWrite  DataStoreName=oPump  DataStoreElements=oPump.oMot_.oState_.oRampDataFluxMasterAngleOffset_.fRampOut_  IndexOptions=Index vector (dialog)  Indices=1  OutputSizes=1
  Data Store Write4 : DataStoreWrite  DataStoreName=oPump  DataStoreElements=oPump.oMot_.oState_.oRampDataFluxMstrAngFrcd2clsdSmoothn_.fSetpoint_  IndexOptions=Index vector (dialog)  Indices=1  OutputSizes=1
  Data Store Write44 : DataStoreWrite  DataStoreName=oPump  DataStoreElements=oPump.oMot_.oState_.oRampDataFluxMasterAngleOffset_.fRampOutDdt_  IndexOptions=Index vector (dialog)  Indices=1  OutputSizes=1
  Data Store Write6 : DataStoreWrite  Commented=on  DataStoreName=oPump  DataStoreElements=oPump.oMot_.oState_.fFluxWeakeningState_  IndexOptions=Index vector (dialog)  Indices=1  OutputSizes=1
  Data Store Write7 : DataStoreWrite  Commented=on  DataStoreName=oPump  DataStoreElements=oPump.oMot_.oState_.oRampDataIdRef_.fSetpoint_  IndexOptions=Index vector (dialog)  Indices=1  OutputSizes=1
  Dynamic Current Limiting Pump : Subsystem  TreatAsAtomicUnit=on
  Equal18 : RelationalOperator  Operator=>  OutDataTypeStr=boolean  RndMeth=Simplest
  Equal19 : RelationalOperator  Operator=>  OutDataTypeStr=boolean  RndMeth=Simplest
  Equal3 : RelationalOperator  Commented=on  Operator=<  OutDataTypeStr=boolean  RndMeth=Simplest
  Gain1 : Gain  Gain=-1
  Max1 : MinMax  Function=max  Inputs=2
  Min : MinMax  Inputs=2
  NOT1 : Logic  Commented=on  Operator=NOT  AllPortsSameDT=off  OutDataTypeStr=boolean
  Scope : Scope  NumInputPorts=3
  Scope1 : Scope  NumInputPorts=2
  Sim Options Prop Id Variant Subsystem : Subsystem  Variant=on
  Sim Options Pump Iq Variant Subsystem : Subsystem  Variant=on
  Sim Options Pump OmegaERef Variant Subsystem : Subsystem  Variant=on
  Subsystem : Subsystem
  Subsystem2 : Subsystem  Commented=on
  Switch23 : Switch  Criteria=u2 > Threshold  Threshold=0.5
  Switch4 : Switch  Criteria=u2 > Threshold
  Switch5 : Switch  Commented=on  Criteria=u2 > Threshold  Threshold=0.5
  Zero11 : Constant  Value=0  OutDataTypeStr=single  SampleTime=-1
  Zero17 : Constant  Value=0.001  OutDataTypeStr=single  SampleTime=-1
  rampStep_oRampDataFluxMasterAngleOffset_ : Reusables_Lib/rampStep_  SystemSampleTime=-1  VariantActivationTime=update diagram  Latency=0  AutoFrameSizeCalculation=off
  rampStep_oRampDataFluxMstrAngFrcd2clsdSmoothn_ : Reusables_Lib/rampStep_  SystemSampleTime=-1  VariantActivationTime=update diagram  Latency=0  AutoFrameSizeCalculation=off
  rampStep_oRampDataIdRef_ : Reusables_Lib/rampStep_  SystemSampleTime=-1  VariantActivationTime=update diagram  Latency=0  AutoFrameSizeCalculation=off
  rampStep_oRampDataIqRef_ : Subsystem  AncestorBlock=Reusables_Lib/rampStep_
  rampStep_oRampDataIqRef_old : Reusables_Lib/rampStep_  Commented=on  SystemSampleTime=-1  VariantActivationTime=update diagram  Latency=0  AutoFrameSizeCalculation=off
  rampStep_oRampDataOmegaERef_ : Reusables_Lib/rampStep_  SystemSampleTime=-1  VariantActivationTime=update diagram  Latency=0  AutoFrameSizeCalculation=off
  wires:
  Data Store Read6/1 -> rampStep_oRampDataIqRef_/5(fRampOut_z)
  Data Store Read71/1 -> rampStep_oRampDataIqRef_/4(fTimestepS_)
  Data Store Read76/1 -> rampStep_oRampDataIqRef_/3(fDDownslope_)
  Data Store Read73/1 -> rampStep_oRampDataIqRef_/2(fUpslope_)
  Sim Options Pump Iq Variant Subsystem/1(fSetpoint_) -> rampStep_oRampDataIqRef_/1(fSetpoint_)
  rampStep_oRampDataIqRef_/1(fRampOut_) -> Data Store Write18/1
  rampStep_oRampDataIqRef_/2(fRampOutDdt_) -> Data Store Write26/1
  Data Store Read15/1 -> rampStep_oRampDataFluxMasterAngleOffset_/2
  Data Store Read4/1 -> rampStep_oRampDataFluxMasterAngleOffset_/1
  rampStep_oRampDataFluxMasterAngleOffset_/2 -> Data Store Write44/1
  Data Store Read64/1 -> rampStep_oRampDataFluxMasterAngleOffset_/4
  rampStep_oRampDataFluxMasterAngleOffset_/1 -> Data Store Write35/1
  Data Store Read63/1 -> rampStep_oRampDataFluxMasterAngleOffset_/3
  Data Store Read5/1 -> Add12/1
  Switch5/1 -> Add12/2
  Subsystem2/1(Out1) -> Switch5/3, Data Store Write6/1
  Constant3/1 -> Switch5/1
  Add12/1 -> Data Store Write7/1
  NOT1/1 -> Subsystem2/Enable
  Equal3/1 -> Switch5/2, NOT1/1
  Abs6/1 -> Equal3/1
  Data Store Read31/1 -> Abs6/1
  Data Store Read65/1 -> Equal3/2
  rampStep_oRampDataFluxMstrAngFrcd2clsdSmoothn_/1 -> Data Store Write2/1
  rampStep_oRampDataFluxMstrAngFrcd2clsdSmoothn_/2 -> Data Store Write3/1
  Data Store Read2/1 -> rampStep_oRampDataFluxMstrAngFrcd2clsdSmoothn_/2
  Zero11/1 -> Data Store Write4/1, rampStep_oRampDataFluxMstrAngFrcd2clsdSmoothn_/1
  Data Store Read1/1 -> rampStep_oRampDataFluxMstrAngFrcd2clsdSmoothn_/4
  Data Store Read3/1 -> rampStep_oRampDataFluxMstrAngFrcd2clsdSmoothn_/3
  Data Store Read78/1 -> rampStep_oRampDataOmegaERef_/2
  Data Store Read87/1 -> rampStep_oRampDataOmegaERef_/3
  Data Store Read62/1 -> Subsystem/Enable
  Data Store Read105/1 -> Scope1/2
  Data Store Read84/1 -> Switch23/1, Equal18/1, Equal19/1
  Data Store Read106/1 -> Scope/3
  rampStep_oRampDataIdRef_/1 -> Data Store Write21/1
  Data Store Read80/1 -> Gain1/1, Min/2
  Data Store Read77/1 -> rampStep_oRampDataOmegaERef_/4
  Equal18/1 -> AND8/1
  Switch23/1 -> Data Store Write19/1  "fIdleCtrlCurrent_"
  Gain1/1 -> Max1/2
  Data Store Read104/1 -> Scope1/1
  Min/1 -> Max1/1
  rampStep_oRampDataOmegaERef_/2 -> Data Store Write27/1
  Data Store Read81/1 -> Dynamic Current Limiting Pump/Enable, Switch4/2
  Switch4/1 -> Equal19/2, Switch23/3
  AND8/1 -> Switch23/2
  rampStep_oRampDataIdRef_/2 -> Data Store Write22/1
  Data Store Read85/1 -> rampStep_oRampDataIdRef_/2
  rampStep_oRampDataOmegaERef_/1 -> Subsystem/1(oRampDataOmegaERef_.fRampOut), Data Store Write23/1
  Data Store Read100/1 -> Scope/2
  Data Store Read10/1 -> Scope/1
  Zero17/1 -> Equal18/2
  Data Store Read82/1 -> Min/1
  Sim Options Prop Id Variant Subsystem/1(Out1) -> rampStep_oRampDataIdRef_/1
  Data Store Read86/1 -> rampStep_oRampDataIdRef_/3
  Sim Options Pump OmegaERef Variant Subsystem/1(Out1) -> rampStep_oRampDataOmegaERef_/1
  Dynamic Current Limiting Pump/1(oRampDataIqRef_.fSetpoint) -> Switch4/1
  Max1/1 -> Switch4/3
  Equal19/1 -> AND8/2
  Data Store Read68/1 -> rampStep_oRampDataIdRef_/4

== system Target_Control_System/Target_Control_System/MainLoop/pumpMotor_mainLoop/motorTaskMainFastStep(&oPump)/Correction Constants for Observer and Control - Pump ==
  note: // ---------------- Correction constants for observer and control ------------
      | 	// Sources of delay:
      | 	//  1. Input.
      | 	//     a) delays from ADCs. Both voltage and current channels use identical ADCs and
      | 	//        initial FPGA processing. The delay on the current channel is taken as a
      | 	//        baseline.
      | 	//
      | 	//     b) Extra delays in the voltage acquisition stage, due to
      | 	//      1) tighter analog filtering
      | 	//      2) the 2 pole LPF filter in the FPGA.
      | 	//
      | 	//  2. Output
      | 	//     a) The PWM duty is updated only once per cycle, causing some delay.
      | 	//        Additionally, the interrupt might be delayed, causing further delays.
      | 	//
      | 	//  3. User specified for testing
      | 	//
      | 	// Values of the above delays:
      | 	//   1.a    A known constant delay is specified for each motor channel. (Mostly driven by the sinc3 filtering.
      |       //            Directly depends on sigma delta frequency.)
      | 	//   1.b.1  A known constant delay is specified for each motor channel
      | 	//   1.b.2  Can be calculated analytically
      | 	//   2.a    Approximated as a constant fraction of the PWM period.
      | 	//
      | 	// Compensation order of the above delays
      | 	//  - The entire interrupt loop runs behind reality by amount 1.a
      | 	//  - The delay on the current acquisition is therefore not compensated at the input to the algorithm.
      | 	//  - The voltage feedback needs to be aligned with the current feedback, and therefore needs to be
      | 	//    corrected for delays 1.b.1 and 1.b.2. This is a phase shift applied to the voltage.
      | 	//  - After the control loop, when the dq quantities are transformed to abc, the remaining delays are
      | 	//    corrected by phase shifting the dq angle. These delays are 1.a, 2.a and 3.
      | 	//
      | 	// Additionally, filter 1.b.2 causes a reduction in amplitude. This is compensated too to ensure
      | 	// a more level flux estimate output at high speeds.
      | 	//
  correctionConstantsObserverControl : TriggerPort  TriggerType=function-call  VariantControl=Variant
  Abs : Abs  OutDataTypeStr=single
  Abs1 : Abs  OutDataTypeStr=single
  Abs4 : Abs  OutDataTypeStr=single
  Add4 : Sum  Inputs=|++
  Add5 : Sum
  AmplitudeRatio : Fcn  Expr=1/sqrt(1+(u*u))
  Atan3 : Trigonometry  Operator=atan2
  Data Store Read14 : DataStoreRead  DataStoreName=oPump  DataStoreElements=oPump.oMot_.oParam_.fIntControlLoopDt_  IndexOptions=Index vector (dialog)  Indices=1  OutputSizes=1
  Data Store Read26 : DataStoreRead  DataStoreName=mdl_pump_fOmegaE  IndexOptions=Index vector (dialog)  Indices=1  OutputSizes=1
  Data Store Read33 : DataStoreRead  DataStoreName=oPump  DataStoreElements=oPump.oMot_.oParam_.fHardwareDelayVoltageAcquisitionExtra_  IndexOptions=Index vector (dialog)  Indices=1  OutputSizes=1
  Data Store Read92 : DataStoreRead  DataStoreName=oPump  DataStoreElements=oPump.oMot_.oParam_.fHardwareDelayCurrentAcquisition_  IndexOptions=Index vector (dialog)  Indices=1  OutputSizes=1
  Data Store Read93 : DataStoreRead  DataStoreName=oPump  DataStoreElements=oPump.oMot_.oParam_.fHardwareDelayControlLoopFraction_  IndexOptions=Index vector (dialog)  Indices=1  OutputSizes=1
  Data Store Write36 : DataStoreWrite  DataStoreName=oPump  DataStoreElements=oPump.oMot_.oState_.oRampDataFluxMasterAngleOffset_.fSetpoint_  IndexOptions=Index vector (dialog)  Indices=1  OutputSizes=1
  Data Store Write4 : DataStoreWrite  DataStoreName=oPump  DataStoreElements=oPump.oMot_.oOut_.fUphFilterAmplitudeRatio_  IndexOptions=Index vector (dialog)  Indices=1  OutputSizes=1
  Data Store Write43 : DataStoreWrite  DataStoreName=oPump  DataStoreElements=oPump.oMot_.oOut_.fUphFilterDelayAngleRad_  IndexOptions=Index vector (dialog)  Indices=1  OutputSizes=1
  Data Store Write8 : DataStoreWrite  DataStoreName=oPump  DataStoreElements=oPump.oMot_.oState_.fOmegaRel_  IndexOptions=Index vector (dialog)  Indices=1  OutputSizes=1
  Gain7 : Gain  Gain=1.414213562
  Product{,5..6,12..13} (5 alike) : Product
  Product1 : Product  OutDataTypeStr=single
  Saturation : Saturate  UpperLimit=inf  LowerLimit=0.3
  Saturation1 : Saturate  UpperLimit=pi/2  LowerLimit=-inf
  Sign : Signum
  Variant Subsystem : Subsystem  Variant=on
  fTemp1 : Fcn  Expr=1-u
  wires:
  Product6/1 -> Data Store Write36/1
  Sign/1 -> Product/2, Product6/1
  Product5/1 -> Product6/2  "fHardwareDelayAngleRad"
  Add5/1 -> Product5/2
  Abs4/1 -> Product5/1
  fTemp1/1 -> Atan3/2
  Data Store Read33/1 -> Product12/2
  Product13/1 -> Add5/2
  Product/1 -> Data Store Write43/1  "fUphFilterDelayAngleRad_"
  Data Store Read14/1 -> Product13/2
  Gain7/1 -> Atan3/1
  Saturation/1 -> Data Store Write4/1  "fUphFilterAmplitudeRatio_"
  Data Store Read26/1 -> Sign/1, Abs4/1, Abs/1  "fOmegaE"
  Saturation1/1 -> Abs1/1
  Add4/1 -> Saturation1/1
  Data Store Read92/1 -> Add5/1
  Variant Subsystem/1(Out1) -> Product1/2, Gain7/1, Product1/1, Data Store Write8/1
  Abs/1 -> Variant Subsystem/1(In1), Product12/1
  AmplitudeRatio/1 -> Saturation/1
  Product1/1 -> AmplitudeRatio/1, fTemp1/1
  Atan3/1 -> Add4/1
  Data Store Read93/1 -> Product13/1
  Abs1/1 -> Product/1
  Product12/1 -> Add4/2
